simulink model "case6"  (R2024b)
settings: Solver=FixedStepAuto  StartTime=0  StopTime=1  FixedStep=1e-7  RelTol=1e-3
values from neighbouring files (symbols this model uses):
  SG_D_1_D = 0.01056    [IEEE9_case_parameters.m]    (also in case1_parameters.m; case2_parameters.m; case3_parameters.m; case4_parameters.m)
  SG_D_1_EnableSaturation = 0    [IEEE9_case_parameters.m]    (also in case1_parameters.m; case2_parameters.m; case3_parameters.m; case4_parameters.m)
  SG_D_1_f0 = 60    [IEEE9_case_parameters.m]    (also in case1_parameters.m; case2_parameters.m; case3_parameters.m; case4_parameters.m)
  SG_D_1_H = 7.5    [IEEE9_case_parameters.m]    (also in case1_parameters.m; case2_parameters.m; case3_parameters.m; case4_parameters.m)
  SG_D_1_K_A = 20    [IEEE9_case_parameters.m]    (also in case1_parameters.m; case2_parameters.m; case3_parameters.m; case4_parameters.m)
  SG_D_1_K_E = 1.000000e+1    (= 10)    [IEEE9_case_parameters.m]    (also in case1_parameters.m; case2_parameters.m; case3_parameters.m; case4_parameters.m)
  SG_D_1_K_F = 2.363    [IEEE9_case_parameters.m]    (also in case1_parameters.m; case2_parameters.m; case3_parameters.m; case4_parameters.m)
  SG_D_1_K_s = 0.5    [IEEE9_case_parameters.m]    (also in case1_parameters.m = 5; case2_parameters.m = 5; case3_parameters.m = 5; case4_parameters.m = 5)
  SG_D_1_R_a = 0.001088    [IEEE9_case_parameters.m]    (also in case1_parameters.m; case2_parameters.m; case3_parameters.m; case4_parameters.m)
  SG_D_1_S_A = 1    [IEEE9_case_parameters.m]    (also in case1_parameters.m; case2_parameters.m; case3_parameters.m; case4_parameters.m)
  SG_D_1_S_B = 0.103    [IEEE9_case_parameters.m]    (also in case1_parameters.m; case2_parameters.m; case3_parameters.m; case4_parameters.m)
  SG_D_1_S_N = 10.659857    [IEEE9_case_parameters.m]    (also in case1_parameters.m; case2_parameters.m; case3_parameters.m; case4_parameters.m)
  SG_D_1_SpeedPara = 200    [IEEE9_case_parameters.m]    (also in case1_parameters.m; case2_parameters.m; case3_parameters.m; case4_parameters.m)
  SG_D_1_T_0 = 0.720173    [IEEE9_case_parameters.m]    (also in case1_parameters.m = 0.755522; case2_parameters.m = 0.808931; case3_parameters.m = 0.869402; case4_parameters.m = 0.729316)
  SG_D_1_T_1 = 0.3    [IEEE9_case_parameters.m]    (also in case1_parameters.m; case2_parameters.m; case3_parameters.m; case4_parameters.m)
  SG_D_1_T_2 = 0.05    [IEEE9_case_parameters.m]    (also in case1_parameters.m; case2_parameters.m; case3_parameters.m; case4_parameters.m)
  SG_D_1_T_3 = 0.02    [IEEE9_case_parameters.m]    (also in case1_parameters.m; case2_parameters.m; case3_parameters.m; case4_parameters.m)
  SG_D_1_T_4 = 0.005    [IEEE9_case_parameters.m]    (also in case1_parameters.m; case2_parameters.m; case3_parameters.m; case4_parameters.m)
  SG_D_1_T_A = 0.02    [IEEE9_case_parameters.m]    (also in case1_parameters.m; case2_parameters.m; case3_parameters.m; case4_parameters.m)
  SG_D_1_T_dd = 8.000000e+0    (= 8)    [IEEE9_case_parameters.m]    (also in case1_parameters.m; case2_parameters.m; case3_parameters.m; case4_parameters.m)
  SG_D_1_T_ddd = 0.04    [IEEE9_case_parameters.m]    (also in case1_parameters.m; case2_parameters.m; case3_parameters.m; case4_parameters.m)
  SG_D_1_T_E = 0.314    [IEEE9_case_parameters.m]    (also in case1_parameters.m; case2_parameters.m; case3_parameters.m; case4_parameters.m)
  SG_D_1_T_F = 0.35    [IEEE9_case_parameters.m]    (also in case1_parameters.m; case2_parameters.m; case3_parameters.m; case4_parameters.m)
  SG_D_1_T_qd = 0.8    [IEEE9_case_parameters.m]    (also in case1_parameters.m; case2_parameters.m; case3_parameters.m; case4_parameters.m)
  SG_D_1_T_qdd = 0.02    [IEEE9_case_parameters.m]    (also in case1_parameters.m; case2_parameters.m; case3_parameters.m; case4_parameters.m)
  SG_D_1_T_speed = 0.1    [IEEE9_case_parameters.m]    (also in case1_parameters.m = 200; case2_parameters.m = 200; case3_parameters.m = 200; case4_parameters.m = 200)
  SG_D_1_T_w = 0.5    [IEEE9_case_parameters.m]    (also in case1_parameters.m; case2_parameters.m; case3_parameters.m; case4_parameters.m)
  SG_D_1_V_ref = 1.990276    [IEEE9_case_parameters.m]    (also in case1_parameters.m = 2.042296; case2_parameters.m = 2.051388; case3_parameters.m = 2.089584; case4_parameters.m = 2.01845)
  SG_D_1_w_ref = 376.991118    [IEEE9_case_parameters.m]    (also in case1_parameters.m; case2_parameters.m; case3_parameters.m; case4_parameters.m)
  SG_D_1_wb = 6.000000e+1    (= 60)    [IEEE9_case_parameters.m]    (also in case1_parameters.m; case2_parameters.m; case3_parameters.m; case4_parameters.m)
  SG_D_1_x_d = 1.9    [IEEE9_case_parameters.m]    (also in case1_parameters.m; case2_parameters.m; case3_parameters.m; case4_parameters.m)
  SG_D_1_x_dd = 0.302    [IEEE9_case_parameters.m]    (also in case1_parameters.m; case2_parameters.m; case3_parameters.m; case4_parameters.m)
  SG_D_1_x_ddd = 0.204    [IEEE9_case_parameters.m]    (also in case1_parameters.m; case2_parameters.m; case3_parameters.m; case4_parameters.m)
  SG_D_1_x_l = 0.05    [IEEE9_case_parameters.m]    (also in case1_parameters.m; case2_parameters.m; case3_parameters.m; case4_parameters.m)
  SG_D_1_x_q = 1.3    [IEEE9_case_parameters.m]    (also in case1_parameters.m; case2_parameters.m; case3_parameters.m; case4_parameters.m)
  SG_D_1_x_qd = 0.5    [IEEE9_case_parameters.m]    (also in case1_parameters.m; case2_parameters.m; case3_parameters.m; case4_parameters.m)
  SG_D_1_x_qdd = 0.3    [IEEE9_case_parameters.m]    (also in case1_parameters.m; case2_parameters.m; case3_parameters.m; case4_parameters.m)
  SG_D_2_D = 0.02    [IEEE9_case_parameters.m]    (also in case1_parameters.m; case2_parameters.m; case3_parameters.m; case4_parameters.m)
  SG_D_2_EnableSaturation = 0    [IEEE9_case_parameters.m]    (also in case1_parameters.m; case2_parameters.m; case3_parameters.m; case4_parameters.m)
  SG_D_2_f0 = 60    [IEEE9_case_parameters.m]    (also in case1_parameters.m; case2_parameters.m; case3_parameters.m; case4_parameters.m)
  SG_D_2_H = 8.000000e+0    (= 8)    [IEEE9_case_parameters.m]    (also in case1_parameters.m; case2_parameters.m; case3_parameters.m; case4_parameters.m)
  SG_D_2_K_A = 20    [IEEE9_case_parameters.m]    (also in case1_parameters.m; case2_parameters.m; case3_parameters.m; case4_parameters.m)
  SG_D_2_K_E = 1.000000e+1    (= 10)    [IEEE9_case_parameters.m]    (also in case1_parameters.m; case2_parameters.m; case3_parameters.m; case4_parameters.m)
  SG_D_2_K_F = 2.363    [IEEE9_case_parameters.m]    (also in case1_parameters.m; case2_parameters.m; case3_parameters.m; case4_parameters.m)
  SG_D_2_K_s = 0.5    [IEEE9_case_parameters.m]    (also in case1_parameters.m = 4; case2_parameters.m = 4; case3_parameters.m = 4; case4_parameters.m = 4)
  SG_D_2_R_a = 0.001088    [IEEE9_case_parameters.m]    (also in case1_parameters.m; case2_parameters.m; case3_parameters.m; case4_parameters.m)
  SG_D_2_S_A = 1    [IEEE9_case_parameters.m]    (also in case1_parameters.m; case2_parameters.m; case3_parameters.m; case4_parameters.m)
  SG_D_2_S_B = 0.103    [IEEE9_case_parameters.m]    (also in case1_parameters.m; case2_parameters.m; case3_parameters.m; case4_parameters.m)
  SG_D_2_S_N = 10.659857    [IEEE9_case_parameters.m]    (also in case1_parameters.m; case2_parameters.m; case3_parameters.m; case4_parameters.m)
  SG_D_2_SpeedPara = 200    [IEEE9_case_parameters.m]    (also in case1_parameters.m; case2_parameters.m; case3_parameters.m; case4_parameters.m)
  SG_D_2_T_0 = 1.632913    [IEEE9_case_parameters.m]    (also in case1_parameters.m = 1.632925; case2_parameters.m = 1.632915; case3_parameters.m = 1.632914; case4_parameters.m = 1.632927)
  SG_D_2_T_1 = 0.2    [IEEE9_case_parameters.m]    (also in case1_parameters.m; case2_parameters.m; case3_parameters.m; case4_parameters.m)
  SG_D_2_T_2 = 0.05    [IEEE9_case_parameters.m]    (also in case1_parameters.m; case2_parameters.m; case3_parameters.m; case4_parameters.m)
  SG_D_2_T_3 = 0.02    [IEEE9_case_parameters.m]    (also in case1_parameters.m; case2_parameters.m; case3_parameters.m; case4_parameters.m)
  SG_D_2_T_4 = 0.005    [IEEE9_case_parameters.m]    (also in case1_parameters.m; case2_parameters.m; case3_parameters.m; case4_parameters.m)
  SG_D_2_T_A = 0.02    [IEEE9_case_parameters.m]    (also in case1_parameters.m; case2_parameters.m; case3_parameters.m; case4_parameters.m)
  SG_D_2_T_dd = 7.9    [IEEE9_case_parameters.m]    (also in case1_parameters.m; case2_parameters.m; case3_parameters.m; case4_parameters.m)
  SG_D_2_T_ddd = 0.04    [IEEE9_case_parameters.m]    (also in case1_parameters.m; case2_parameters.m; case3_parameters.m; case4_parameters.m)
  SG_D_2_T_E = 0.314    [IEEE9_case_parameters.m]    (also in case1_parameters.m; case2_parameters.m; case3_parameters.m; case4_parameters.m)
  SG_D_2_T_F = 0.35    [IEEE9_case_parameters.m]    (also in case1_parameters.m; case2_parameters.m; case3_parameters.m; case4_parameters.m)
  SG_D_2_T_qd = 0.8    [IEEE9_case_parameters.m]    (also in case1_parameters.m; case2_parameters.m; case3_parameters.m; case4_parameters.m)
  SG_D_2_T_qdd = 0.015    [IEEE9_case_parameters.m]    (also in case1_parameters.m; case2_parameters.m; case3_parameters.m; case4_parameters.m)
  SG_D_2_T_speed = 0.1    [IEEE9_case_parameters.m]    (also in case1_parameters.m = 150; case2_parameters.m = 150; case3_parameters.m = 150; case4_parameters.m = 150)
  SG_D_2_T_w = 0.35    [IEEE9_case_parameters.m]    (also in case1_parameters.m; case2_parameters.m; case3_parameters.m; case4_parameters.m)
  SG_D_2_V_ref = 2.58547    [IEEE9_case_parameters.m]    (also in case1_parameters.m = 2.597896; case2_parameters.m = 2.587136; case3_parameters.m = 2.586042; case4_parameters.m = 2.599679)
  SG_D_2_w_ref = 376.991118    [IEEE9_case_parameters.m]    (also in case1_parameters.m; case2_parameters.m; case3_parameters.m; case4_parameters.m)
  SG_D_2_wb = 6.000000e+1    (= 60)    [IEEE9_case_parameters.m]    (also in case1_parameters.m; case2_parameters.m; case3_parameters.m; case4_parameters.m)
  SG_D_2_x_d = 1.8    [IEEE9_case_parameters.m]    (also in case1_parameters.m; case2_parameters.m; case3_parameters.m; case4_parameters.m)
  SG_D_2_x_dd = 0.302    [IEEE9_case_parameters.m]    (also in case1_parameters.m; case2_parameters.m; case3_parameters.m; case4_parameters.m)
  SG_D_2_x_ddd = 0.204    [IEEE9_case_parameters.m]    (also in case1_parameters.m; case2_parameters.m; case3_parameters.m; case4_parameters.m)
  SG_D_2_x_l = 0.05    [IEEE9_case_parameters.m]    (also in case1_parameters.m; case2_parameters.m; case3_parameters.m; case4_parameters.m)
  SG_D_2_x_q = 1.25    [IEEE9_case_parameters.m]    (also in case1_parameters.m; case2_parameters.m; case3_parameters.m; case4_parameters.m)
  SG_D_2_x_qd = 0.5    [IEEE9_case_parameters.m]    (also in case1_parameters.m; case2_parameters.m; case3_parameters.m; case4_parameters.m)
  SG_D_2_x_qdd = 0.3    [IEEE9_case_parameters.m]    (also in case1_parameters.m; case2_parameters.m; case3_parameters.m; case4_parameters.m)
  SG_D_3_D = 0.02    [IEEE9_case_parameters.m]    (also in case1_parameters.m; case2_parameters.m; case3_parameters.m; case4_parameters.m)
  SG_D_3_EnableSaturation = 0    [IEEE9_case_parameters.m]    (also in case1_parameters.m; case2_parameters.m; case3_parameters.m; case4_parameters.m)
  SG_D_3_f0 = 60    [IEEE9_case_parameters.m]    (also in case1_parameters.m; case2_parameters.m; case3_parameters.m; case4_parameters.m)
  SG_D_3_H = 7.7    [IEEE9_case_parameters.m]    (also in case1_parameters.m; case2_parameters.m; case3_parameters.m; case4_parameters.m)
  SG_D_3_K_A = 20    [IEEE9_case_parameters.m]    (also in case1_parameters.m; case2_parameters.m; case3_parameters.m; case4_parameters.m)
  SG_D_3_K_E = 1.000000e+1    (= 10)    [IEEE9_case_parameters.m]    (also in case1_parameters.m; case2_parameters.m; case3_parameters.m; case4_parameters.m)
  SG_D_3_K_F = 2.363    [IEEE9_case_parameters.m]    (also in case1_parameters.m; case2_parameters.m; case3_parameters.m; case4_parameters.m)
  SG_D_3_K_s = 0.2    [IEEE9_case_parameters.m]    (also in case1_parameters.m = 2; case2_parameters.m = 2; case3_parameters.m = 2; case4_parameters.m = 2)
  SG_D_3_R_a = 0.001088    [IEEE9_case_parameters.m]    (also in case1_parameters.m; case2_parameters.m; case3_parameters.m; case4_parameters.m)
  SG_D_3_S_A = 1    [IEEE9_case_parameters.m]    (also in case1_parameters.m; case2_parameters.m; case3_parameters.m; case4_parameters.m)
  SG_D_3_S_B = 0.103    [IEEE9_case_parameters.m]    (also in case1_parameters.m; case2_parameters.m; case3_parameters.m; case4_parameters.m)
  SG_D_3_S_N = 10.659857    [IEEE9_case_parameters.m]    (also in case1_parameters.m; case2_parameters.m; case3_parameters.m; case4_parameters.m)
  SG_D_3_SpeedPara = 200    [IEEE9_case_parameters.m]    (also in case1_parameters.m; case2_parameters.m; case3_parameters.m; case4_parameters.m)
  SG_D_3_T_0 = 0.850788    [IEEE9_case_parameters.m]    (also in case1_parameters.m = 0.850786; case2_parameters.m = 0.850787; case3_parameters.m; case4_parameters.m = 0.850786)
  SG_D_3_T_1 = 0.2    [IEEE9_case_parameters.m]    (also in case1_parameters.m; case2_parameters.m; case3_parameters.m; case4_parameters.m)
  SG_D_3_T_2 = 0.05    [IEEE9_case_parameters.m]    (also in case1_parameters.m; case2_parameters.m; case3_parameters.m; case4_parameters.m)
  SG_D_3_T_3 = 0.02    [IEEE9_case_parameters.m]    (also in case1_parameters.m; case2_parameters.m; case3_parameters.m; case4_parameters.m)
  SG_D_3_T_4 = 0.005    [IEEE9_case_parameters.m]    (also in case1_parameters.m; case2_parameters.m; case3_parameters.m; case4_parameters.m)
  SG_D_3_T_A = 0.02    [IEEE9_case_parameters.m]    (also in case1_parameters.m; case2_parameters.m; case3_parameters.m; case4_parameters.m)
  SG_D_3_T_dd = 8.1    [IEEE9_case_parameters.m]    (also in case1_parameters.m; case2_parameters.m; case3_parameters.m; case4_parameters.m)
  SG_D_3_T_ddd = 0.04    [IEEE9_case_parameters.m]    (also in case1_parameters.m; case2_parameters.m; case3_parameters.m; case4_parameters.m)
  SG_D_3_T_E = 0.314    [IEEE9_case_parameters.m]    (also in case1_parameters.m; case2_parameters.m; case3_parameters.m; case4_parameters.m)
  SG_D_3_T_F = 0.35    [IEEE9_case_parameters.m]    (also in case1_parameters.m; case2_parameters.m; case3_parameters.m; case4_parameters.m)
  SG_D_3_T_qd = 0.8    [IEEE9_case_parameters.m]    (also in case1_parameters.m; case2_parameters.m; case3_parameters.m; case4_parameters.m)
  SG_D_3_T_qdd = 0.015    [IEEE9_case_parameters.m]    (also in case1_parameters.m; case2_parameters.m; case3_parameters.m; case4_parameters.m)
  SG_D_3_T_speed = 0.1    [IEEE9_case_parameters.m]    (also in case1_parameters.m = 180; case2_parameters.m = 180; case3_parameters.m = 180; case4_parameters.m = 180)
  SG_D_3_T_w = 0.4    [IEEE9_case_parameters.m]    (also in case1_parameters.m; case2_parameters.m; case3_parameters.m; case4_parameters.m)
  SG_D_3_V_ref = 1.892727    [IEEE9_case_parameters.m]    (also in case1_parameters.m = 1.906439; case2_parameters.m = 1.895535; case3_parameters.m = 1.892105; case4_parameters.m = 1.906598)
  SG_D_3_w_ref = 376.991118    [IEEE9_case_parameters.m]    (also in case1_parameters.m; case2_parameters.m; case3_parameters.m; case4_parameters.m)
  SG_D_3_wb = 6.000000e+1    (= 60)    [IEEE9_case_parameters.m]    (also in case1_parameters.m; case2_parameters.m; case3_parameters.m; case4_parameters.m)
  SG_D_3_x_d = 1.85    [IEEE9_case_parameters.m]    (also in case1_parameters.m; case2_parameters.m; case3_parameters.m; case4_parameters.m)
  SG_D_3_x_dd = 0.302    [IEEE9_case_parameters.m]    (also in case1_parameters.m; case2_parameters.m; case3_parameters.m; case4_parameters.m)
  SG_D_3_x_ddd = 0.204    [IEEE9_case_parameters.m]    (also in case1_parameters.m; case2_parameters.m; case3_parameters.m; case4_parameters.m)
  SG_D_3_x_l = 0.05    [IEEE9_case_parameters.m]    (also in case1_parameters.m; case2_parameters.m; case3_parameters.m; case4_parameters.m)
  SG_D_3_x_q = 1.2    [IEEE9_case_parameters.m]    (also in case1_parameters.m; case2_parameters.m; case3_parameters.m; case4_parameters.m)
  SG_D_3_x_qd = 0.5    [IEEE9_case_parameters.m]    (also in case1_parameters.m; case2_parameters.m; case3_parameters.m; case4_parameters.m)
  SG_D_3_x_qdd = 0.3    [IEEE9_case_parameters.m]    (also in case1_parameters.m; case2_parameters.m; case3_parameters.m; case4_parameters.m)
(part 11 of 12)

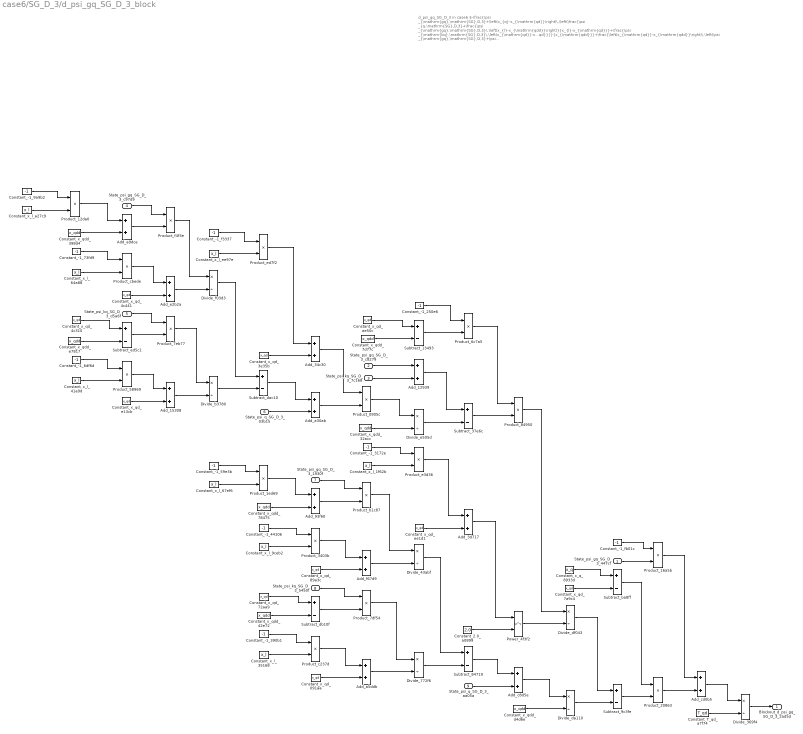
== system case6/SG_D_3/d_psi_gq_SG_D_3_block ==
  note: d_psi_gq_SG_D_3 in case6
      | $-\frac{\psi _{\mathrm{gq},\mathrm{SG},D,3}+\left(x_{q}-x_{\mathrm{qd}}\right)\,\left(\frac{\psi _{q,\mathrm{SG},D,3}+\frac{\psi _{\mathrm{gq},\mathrm{SG},D,3}\,\left(x_{l}-x_{\mathrm{qdd}}\right)}{x_{l}-x_{\mathrm{qd}}}+\frac{\psi _{\mathrm{kq},\mathrm{SG},D,3}\,\left(x_{\mathrm{qd}}-x_{\mathrm{qdd}}\right)}{x_{l}-x_{\mathrm{qd}}}}{x_{\mathrm{qdd}}}+\frac{\left(x_{\mathrm{qd}}-x_{\mathrm{qdd}}\right)\,\left(\psi _{\mathrm{gq},\mathrm{SG},D,3}+\psi _{\mathrm{kq},\mathrm{SG},D,3}+\frac{\left(x_{l}-x_{\mathrm{qd}}\right)\,\left(\psi _{q,\mathrm{SG},D,3}+\frac{\psi _{\mathrm{gq},\mathrm{SG},D,3}\,\left(x_{l}-x_{\mathrm{qdd}}\right)}{x_{l}-x_{\mathrm{qd}}}+\frac{\psi _{\mathrm{kq},\mathrm{SG},D,3}\,\left(x_{\mathrm{qd}}-x_{\mathrm{qdd}}\right)}{x_{l}-x_{\mathrm{qd}}}\right)}{x_{\mathrm{qdd}}}\right)}{{\left(x_{l}-x_{\mathrm{qd}}\right)}^2}\right)}{T_{\mathrm{qd}}}$
      | Automatically generated on 2025-10-31 19:19:17 .
  State_psi_gq_SG_D_3_447cf : Inport
  State_psi_gq_SG_D_3_c8279 : Inport  Port=2
  State_psi_kq_SG_D_3_7c168 : Inport  Port=3
  State_psi_gq_SG_D_3_c97d9 : Inport  Port=4
  State_psi_kq_SG_D_3_d5a6f : Inport  Port=5
  State_psi_q_SG_D_3_03b15 : Inport  Port=6
  State_psi_gq_SG_D_3_1930f : Inport  Port=7
  State_psi_kq_SG_D_3_5450f : Inport  Port=8
  State_psi_q_SG_D_3_aa05a : Inport  Port=9
  Add_12939 : Sum
  Add_15308 : Sum
  Add_34c30 : Sum
  Add_3d717 : Sum
  Add_93f60 : Sum
  Add_a30ab : Sum
  Add_a5ddb : Sum
  Add_a9dce : Sum
  Add_c8d5e : Sum
  Add_cd0b5 : Sum
  Add_e2b2a : Sum
  Add_f67d9 : Sum
  Constant_-1_250e6 : Constant  Value=-1
  Constant_-1_3172e : Constant  Value=-1
  Constant_-1_390b1 : Constant  Value=-1
  Constant_-1_44106 : Constant  Value=-1
  Constant_-1_59e3b : Constant  Value=-1
  Constant_-1_6df6d : Constant  Value=-1
  Constant_-1_73fd9 : Constant  Value=-1
  Constant_-1_9a9b2 : Constant  Value=-1
  Constant_-1_f3337 : Constant  Value=-1
  Constant_-1_fb01c : Constant  Value=-1
  Constant_2.0_a0899 : Constant  Value=2.0
  Constant_T_qd_a7f74 : Constant  Value=T_qd
  Constant_x_l_1f62b : Constant  Value=x_l
  Constant_x_l_35168 : Constant  Value=x_l
  Constant_x_l_41a9d : Constant  Value=x_l
  Constant_x_l_64a88 : Constant  Value=x_l
  Constant_x_l_67ef6 : Constant  Value=x_l
  Constant_x_l_9ceb2 : Constant  Value=x_l
  Constant_x_l_a27c9 : Constant  Value=x_l
  Constant_x_l_ee97e : Constant  Value=x_l
  Constant_x_q_8933d : Constant  Value=x_q
  Constant_x_qd_091aa : Constant  Value=x_qd
  Constant_x_qd_3e35b : Constant  Value=x_qd
  Constant_x_qd_4c310 : Constant  Value=x_qd
  Constant_x_qd_4c441 : Constant  Value=x_qd
  Constant_x_qd_72aa9 : Constant  Value=x_qd
  Constant_x_qd_7a9c4 : Constant  Value=x_qd
  Constant_x_qd_89a3c : Constant  Value=x_qd
  Constant_x_qd_ae50c : Constant  Value=x_qd
  Constant_x_qd_e13cb : Constant  Value=x_qd
  Constant_x_qd_ee1d1 : Constant  Value=x_qd
  Constant_x_qdd_32acc : Constant  Value=x_qdd
  Constant_x_qdd_398d4 : Constant  Value=x_qdd
  Constant_x_qdd_42e72 : Constant  Value=x_qdd
  Constant_x_qdd_78475 : Constant  Value=x_qdd
  Constant_x_qdd_7d77c : Constant  Value=x_qdd
  Constant_x_qdd_d4d6e : Constant  Value=x_qdd
  Constant_x_qdd_e7817 : Constant  Value=x_qdd
  Divide_369f4 : Product  Inputs=*/
  Divide_43abf : Product  Inputs=*/
  Divide_772f6 : Product  Inputs=*/
  Divide_b3780 : Product  Inputs=*/
  Divide_da110 : Product  Inputs=*/
  Divide_df043 : Product  Inputs=*/
  Divide_e505d : Product  Inputs=*/
  Divide_f03d3 : Product  Inputs=*/
  Power_4f3f2 : Math  Operator=pow
  Product_0905c : Product
  Product_12da0 : Product
  Product_16a5b : Product
  Product_1ed69 : Product
  Product_20863 : Product
  Product_3403b : Product
  Product_58969 : Product
  Product_6c7a5 : Product
  Product_7df54 : Product
  Product_7eb77 : Product
  Product_84950 : Product
  Product_b1c87 : Product
  Product_c237d : Product
  Product_cbede : Product
  Product_e3d36 : Product
  Product_ed7f2 : Product
  Product_f4f3e : Product
  Subtract_13493 : Sum  Inputs=+-
  Subtract_37e6c : Sum  Inputs=+-
  Subtract_84719 : Sum  Inputs=+-
  Subtract_9c3fe : Sum  Inputs=+-
  Subtract_ba8ff : Sum  Inputs=+-
  Subtract_dac10 : Sum  Inputs=+-
  Subtract_db10f : Sum  Inputs=+-
  Subtract_ed5c1 : Sum  Inputs=+-
  Blockout_d_psi_gq_SG_D_3_2ad5d : Outport
  wires:
  Constant_x_l_1f62b/1 -> Product_e3d36/2
  Constant_x_qd_4c310/1 -> Subtract_ed5c1/1
  Add_34c30/1 -> Product_0905c/1
  Constant_-1_9a9b2/1 -> Product_12da0/1
  Add_a9dce/1 -> Product_f4f3e/2
  Constant_x_qdd_e7817/1 -> Subtract_ed5c1/2
  Constant_x_qd_3e35b/1 -> Add_34c30/2
  Constant_x_l_a27c9/1 -> Product_12da0/2
  Constant_x_l_64a88/1 -> Product_cbede/2
  Add_a5ddb/1 -> Divide_772f6/2
  State_psi_kq_SG_D_3_7c168/1 -> Add_12939/2
  Constant_x_qdd_398d4/1 -> Add_a9dce/2
  Product_12da0/1 -> Add_a9dce/1
  Constant_x_qd_091aa/1 -> Add_a5ddb/2
  Product_6c7a5/1 -> Product_84950/1
  Constant_-1_59e3b/1 -> Product_1ed69/1
  Constant_-1_73fd9/1 -> Product_cbede/1
  Constant_-1_6df6d/1 -> Product_58969/1
  Constant_x_l_41a9d/1 -> Product_58969/2
  Constant_-1_250e6/1 -> Product_6c7a5/1
  Constant_-1_fb01c/1 -> Product_16a5b/1
  State_psi_gq_SG_D_3_c97d9/1 -> Product_f4f3e/1
  Product_1ed69/1 -> Add_93f60/1
  Product_cbede/1 -> Add_e2b2a/1
  Product_c237d/1 -> Add_a5ddb/1
  Constant_x_qd_4c441/1 -> Add_e2b2a/2
  Constant_-1_44106/1 -> Product_3403b/1
  State_psi_kq_SG_D_3_d5a6f/1 -> Product_7eb77/1
  Subtract_ed5c1/1 -> Product_7eb77/2
  Product_58969/1 -> Add_15308/1
  Add_93f60/1 -> Product_b1c87/2
  Add_e2b2a/1 -> Divide_f03d3/2
  Constant_x_qd_e13cb/1 -> Add_15308/2
  Product_f4f3e/1 -> Divide_f03d3/1
  Constant_T_qd_a7f74/1 -> Divide_369f4/2
  Product_3403b/1 -> Add_f67d9/1
  Product_7eb77/1 -> Divide_b3780/1
  Product_7df54/1 -> Divide_772f6/1
  Add_15308/1 -> Divide_b3780/2
  Constant_-1_f3337/1 -> Product_ed7f2/1
  Constant_x_qdd_32acc/1 -> Divide_e505d/2
  Constant_x_l_ee97e/1 -> Product_ed7f2/2
  Divide_f03d3/1 -> Subtract_dac10/1
  Constant_x_qd_7a9c4/1 -> Subtract_ba8ff/2
  Add_f67d9/1 -> Divide_43abf/2
  Divide_b3780/1 -> Subtract_dac10/2
  Constant_x_l_67ef6/1 -> Product_1ed69/2
  Product_ed7f2/1 -> Add_34c30/1
  Constant_-1_3172e/1 -> Product_e3d36/1
  Constant_x_l_9ceb2/1 -> Product_3403b/2
  Subtract_dac10/1 -> Add_a30ab/1
  State_psi_q_SG_D_3_03b15/1 -> Add_a30ab/2
  Constant_-1_390b1/1 -> Product_c237d/1
  Constant_x_qdd_78475/1 -> Add_93f60/2
  Constant_x_qd_72aa9/1 -> Subtract_db10f/1
  Constant_x_qdd_42e72/1 -> Subtract_db10f/2
  Constant_x_l_35168/1 -> Product_c237d/2
  Add_a30ab/1 -> Product_0905c/2
  Constant_x_qdd_7d77c/1 -> Subtract_13493/2
  State_psi_gq_SG_D_3_1930f/1 -> Product_b1c87/1
  Constant_x_qd_89a3c/1 -> Add_f67d9/2
  Divide_df043/1 -> Subtract_9c3fe/1
  State_psi_kq_SG_D_3_5450f/1 -> Product_7df54/1
  Subtract_db10f/1 -> Product_7df54/2
  Constant_x_qd_ae50c/1 -> Subtract_13493/1
  State_psi_gq_SG_D_3_c8279/1 -> Add_12939/1
  Product_0905c/1 -> Divide_e505d/1
  Product_b1c87/1 -> Divide_43abf/1
  Subtract_13493/1 -> Product_6c7a5/2
  Add_12939/1 -> Subtract_37e6c/1
  Divide_e505d/1 -> Subtract_37e6c/2
  Product_e3d36/1 -> Add_3d717/1
  Constant_x_qd_ee1d1/1 -> Add_3d717/2
  Divide_43abf/1 -> Subtract_84719/1
  Divide_772f6/1 -> Subtract_84719/2
  Subtract_37e6c/1 -> Product_84950/2
  Add_3d717/1 -> Power_4f3f2/1
  Constant_2.0_a0899/1 -> Power_4f3f2/2
  Subtract_84719/1 -> Add_c8d5e/1
  State_psi_q_SG_D_3_aa05a/1 -> Add_c8d5e/2
  Product_84950/1 -> Divide_df043/1
  Power_4f3f2/1 -> Divide_df043/2
  Add_c8d5e/1 -> Divide_da110/1
  Constant_x_qdd_d4d6e/1 -> Divide_da110/2
  Constant_x_q_8933d/1 -> Subtract_ba8ff/1
  Divide_da110/1 -> Subtract_9c3fe/2
  State_psi_gq_SG_D_3_447cf/1 -> Product_16a5b/2
  Subtract_ba8ff/1 -> Product_20863/1
  Subtract_9c3fe/1 -> Product_20863/2
  Product_16a5b/1 -> Add_cd0b5/1
  Product_20863/1 -> Add_cd0b5/2
  Add_cd0b5/1 -> Divide_369f4/1
  Divide_369f4/1 -> Blockout_d_psi_gq_SG_D_3_2ad5d/1

== system case6/SG_D_3/d_psi_kq_SG_D_3_block ==
  note: d_psi_kq_SG_D_3 in case6
      | $-\frac{\psi _{\mathrm{gq},\mathrm{SG},D,3}+\psi _{\mathrm{kq},\mathrm{SG},D,3}+\frac{\left(x_{l}-x_{\mathrm{qd}}\right)\,\left(\psi _{q,\mathrm{SG},D,3}+\frac{\psi _{\mathrm{gq},\mathrm{SG},D,3}\,\left(x_{l}-x_{\mathrm{qdd}}\right)}{x_{l}-x_{\mathrm{qd}}}+\frac{\psi _{\mathrm{kq},\mathrm{SG},D,3}\,\left(x_{\mathrm{qd}}-x_{\mathrm{qdd}}\right)}{x_{l}-x_{\mathrm{qd}}}\right)}{x_{\mathrm{qdd}}}}{T_{\mathrm{qdd}}}$
      | Automatically generated on 2025-10-31 19:19:21 .
  State_psi_gq_SG_D_3_3c968 : Inport
  State_psi_kq_SG_D_3_3550c : Inport  Port=2
  State_psi_gq_SG_D_3_f59cb : Inport  Port=3
  State_psi_kq_SG_D_3_48ef7 : Inport  Port=4
  State_psi_q_SG_D_3_2ea7c : Inport  Port=5
  Add_13628 : Sum
  Add_20637 : Sum
  Add_9f267 : Sum
  Add_a93cc : Sum
  Add_beb3e : Sum
  Add_d8732 : Sum
  Constant_-1_156e6 : Constant  Value=-1
  Constant_-1_5e9c5 : Constant  Value=-1
  Constant_-1_91f7a : Constant  Value=-1
  Constant_-1_da3ff : Constant  Value=-1
  Constant_-1_f171e : Constant  Value=-1
  Constant_T_qdd_c61c0 : Constant  Value=T_qdd
  Constant_x_l_1047d : Constant  Value=x_l
  Constant_x_l_3ae0a : Constant  Value=x_l
  Constant_x_l_9f8e8 : Constant  Value=x_l
  Constant_x_l_b4688 : Constant  Value=x_l
  Constant_x_qd_0905a : Constant  Value=x_qd
  Constant_x_qd_132c0 : Constant  Value=x_qd
  Constant_x_qd_4efa9 : Constant  Value=x_qd
  Constant_x_qd_d7acd : Constant  Value=x_qd
  Constant_x_qdd_76578 : Constant  Value=x_qdd
  Constant_x_qdd_b57e8 : Constant  Value=x_qdd
  Constant_x_qdd_babf2 : Constant  Value=x_qdd
  Divide_10821 : Product  Inputs=*/
  Divide_59c15 : Product  Inputs=*/
  Divide_b33fe : Product  Inputs=*/
  Divide_e3776 : Product  Inputs=*/
  Product_13363 : Product
  Product_4261e : Product
  Product_59fdc : Product
  Product_92618 : Product
  Product_b511d : Product
  Product_e2e02 : Product
  Product_e47ab : Product
  Product_faf11 : Product
  Subtract_0efec : Sum  Inputs=+-
  Subtract_c2b4a : Sum  Inputs=+-
  Subtract_f68ea : Sum  Inputs=+-
  Blockout_d_psi_kq_SG_D_3_6fe0f : Outport
  wires:
  State_psi_q_SG_D_3_2ea7c/1 -> Add_13628/2
  Constant_-1_5e9c5/1 -> Product_b511d/1
  Constant_-1_156e6/1 -> Product_4261e/1
  Constant_-1_f171e/1 -> Product_13363/1
  Constant_x_l_1047d/1 -> Product_b511d/2
  Constant_x_qdd_babf2/1 -> Add_a93cc/2
  Product_e2e02/1 -> Add_20637/1
  Constant_x_l_3ae0a/1 -> Product_4261e/2
  Constant_x_qd_0905a/1 -> Subtract_c2b4a/1
  Product_4261e/1 -> Add_a93cc/1
  Constant_x_l_9f8e8/1 -> Product_92618/2
  Constant_x_qdd_76578/1 -> Subtract_c2b4a/2
  Constant_-1_da3ff/1 -> Product_e2e02/1
  Constant_x_l_b4688/1 -> Product_e2e02/2
  State_psi_gq_SG_D_3_f59cb/1 -> Product_faf11/1
  Add_a93cc/1 -> Product_faf11/2
  Add_13628/1 -> Product_59fdc/2
  Product_b511d/1 -> Add_d8732/1
  Constant_x_qd_132c0/1 -> Add_d8732/2
  State_psi_kq_SG_D_3_48ef7/1 -> Product_e47ab/1
  Subtract_c2b4a/1 -> Product_e47ab/2
  Add_d8732/1 -> Divide_b33fe/2
  Constant_x_qd_d7acd/1 -> Add_20637/2
  Product_faf11/1 -> Divide_b33fe/1
  Product_e47ab/1 -> Divide_10821/1
  Add_20637/1 -> Divide_10821/2
  Constant_-1_91f7a/1 -> Product_92618/1
  Divide_b33fe/1 -> Subtract_0efec/1
  Add_9f267/1 -> Divide_e3776/1
  Divide_10821/1 -> Subtract_0efec/2
  Divide_e3776/1 -> Blockout_d_psi_kq_SG_D_3_6fe0f/1
  Product_92618/1 -> Add_beb3e/1
  Constant_x_qd_4efa9/1 -> Add_beb3e/2
  Subtract_0efec/1 -> Add_13628/1
  State_psi_gq_SG_D_3_3c968/1 -> Product_13363/2
  Add_beb3e/1 -> Product_59fdc/1
  Constant_T_qdd_c61c0/1 -> Divide_e3776/2
  Product_13363/1 -> Subtract_f68ea/1
  State_psi_kq_SG_D_3_3550c/1 -> Subtract_f68ea/2
  Product_59fdc/1 -> Divide_59c15/1
  Constant_x_qdd_b57e8/1 -> Divide_59c15/2
  Subtract_f68ea/1 -> Add_9f267/1
  Divide_59c15/1 -> Add_9f267/2

== system case6/SG_D_3/d_psi_q_SG_D_3_block ==
  note: d_psi_q_SG_D_3 in case6
      | $2\,\pi \,f_{0}\,\left(v_{d,\mathrm{SG},D,3}\,\cos\left(\theta _{\mathrm{SG},D,3}\right)+v_{q,\mathrm{SG},D,3}\,\sin\left(\theta _{\mathrm{SG},D,3}\right)-\frac{R_{a}\,\left(\psi _{q,\mathrm{SG},D,3}+\frac{\psi _{\mathrm{gq},\mathrm{SG},D,3}\,\left(x_{l}-x_{\mathrm{qdd}}\right)}{x_{l}-x_{\mathrm{qd}}}+\frac{\psi _{\mathrm{kq},\mathrm{SG},D,3}\,\left(x_{\mathrm{qd}}-x_{\mathrm{qdd}}\right)}{x_{l}-x_{\mathrm{qd}}}\right)}{x_{\mathrm{qdd}}}-\frac{\psi _{d,\mathrm{SG},D,3}\,w_{\mathrm{SG},D,3}}{2\,f_{0}\,\pi }\right)$
      | Automatically generated on 2025-10-31 19:18:59 .
  State_psi_gq_SG_D_3_44472 : Inport
  State_psi_kq_SG_D_3_a31f2 : Inport  Port=2
  State_psi_q_SG_D_3_3f014 : Inport  Port=3
  Input_v_d_SG_D_3_e9461 : Inport  Port=4
  State_theta_SG_D_3_3efc2 : Inport  Port=5
  Input_v_q_SG_D_3_d5a90 : Inport  Port=6
  State_theta_SG_D_3_e3679 : Inport  Port=7
  State_psi_d_SG_D_3_960b3 : Inport  Port=8
  State_w_SG_D_3_8c018 : Inport  Port=9
  Add_02d73 : Sum
  Add_3103c : Sum
  Add_8a7a6 : Sum
  Add_b9382 : Sum
  Add_c36db : Sum
  Constant_-1_739e7 : Constant  Value=-1
  Constant_-1_b34a5 : Constant  Value=-1
  Constant_-1_e5c6c : Constant  Value=-1
  Constant_-2.0_83048 : Constant  Value=-2.0
  Constant_2.0_3fe72 : Constant  Value=2.0
  Constant_R_a_d1c7d : Constant  Value=R_a
  Constant_f0_02d55 : Constant  Value=f0
  Constant_f0_054a1 : Constant  Value=f0
  Constant_pi_7d6a3 : Constant  Value=pi
  Constant_pi_ed56b : Constant  Value=pi
  Constant_x_l_15983 : Constant  Value=x_l
  Constant_x_l_3eb4b : Constant  Value=x_l
  Constant_x_l_daef7 : Constant  Value=x_l
  Constant_x_qd_65832 : Constant  Value=x_qd
  Constant_x_qd_7332c : Constant  Value=x_qd
  Constant_x_qd_b3384 : Constant  Value=x_qd
  Constant_x_qdd_1628b : Constant  Value=x_qdd
  Constant_x_qdd_341ac : Constant  Value=x_qdd
  Constant_x_qdd_f3557 : Constant  Value=x_qdd
  Divide_1b0b8 : Product  Inputs=*/
  Divide_28c9d : Product  Inputs=*/
  Divide_39289 : Product  Inputs=*/
  Divide_aa057 : Product  Inputs=*/
  MathFunc_cos_f9ceb : Trigonometry  Operator=cos
  MathFunc_sin_8cffe : Trigonometry
  Product_262db : Product
  Product_4ef78 : Product
  Product_5c219 : Product
  Product_6bef6 : Product
  Product_76210 : Product
  Product_82413 : Product
  Product_c6627 : Product
  Product_cbe64 : Product
  Product_cd56f : Product
  Product_d3a60 : Product
  Product_d4924 : Product
  Product_d9336 : Product
  Product_f5a51 : Product
  Product_fddf4 : Product
  Subtract_1f664 : Sum  Inputs=+-
  Subtract_2575a : Sum  Inputs=+-
  Subtract_55639 : Sum  Inputs=+-
  Subtract_e78ca : Sum  Inputs=+-
  Blockout_d_psi_q_SG_D_3_c3e35 : Outport
  wires:
  Constant_x_qd_7332c/1 -> Subtract_e78ca/1
  Constant_pi_7d6a3/1 -> Product_4ef78/2
  Product_76210/1 -> Divide_1b0b8/1
  Constant_x_l_15983/1 -> Product_6bef6/2
  Constant_f0_02d55/1 -> Product_d9336/2
  State_w_SG_D_3_8c018/1 -> Product_cbe64/2
  Constant_-1_b34a5/1 -> Product_82413/1
  Constant_x_qdd_1628b/1 -> Add_c36db/2
  Input_v_d_SG_D_3_e9461/1 -> Product_5c219/1
  Constant_x_qdd_f3557/1 -> Subtract_e78ca/2
  Constant_x_l_3eb4b/1 -> Product_82413/2
  Divide_39289/1 -> Add_02d73/2
  Product_82413/1 -> Add_c36db/1
  Constant_2.0_3fe72/1 -> Product_4ef78/1
  Add_b9382/1 -> Product_76210/2
  Constant_-1_739e7/1 -> Product_6bef6/1
  Constant_x_qd_b3384/1 -> Add_8a7a6/2
  Constant_-1_e5c6c/1 -> Product_f5a51/1
  Subtract_55639/1 -> Subtract_2575a/1
  Constant_x_l_daef7/1 -> Product_f5a51/2
  Subtract_2575a/1 -> Add_02d73/1
  Constant_f0_054a1/1 -> Product_cd56f/2
  State_theta_SG_D_3_e3679/1 -> MathFunc_sin_8cffe/1
  Constant_x_qd_65832/1 -> Add_3103c/2
  State_psi_gq_SG_D_3_44472/1 -> Product_fddf4/1
  Add_c36db/1 -> Product_fddf4/2
  Product_4ef78/1 -> Product_cd56f/1
  Product_6bef6/1 -> Add_3103c/1
  State_psi_kq_SG_D_3_a31f2/1 -> Product_d4924/1
  Subtract_e78ca/1 -> Product_d4924/2
  Product_f5a51/1 -> Add_8a7a6/1
  MathFunc_sin_8cffe/1 -> Product_d3a60/2
  Product_fddf4/1 -> Divide_28c9d/1
  Product_cd56f/1 -> Divide_39289/2
  Add_3103c/1 -> Divide_28c9d/2
  Product_d4924/1 -> Divide_aa057/1
  Add_8a7a6/1 -> Divide_aa057/2
  Input_v_q_SG_D_3_d5a90/1 -> Product_d3a60/1
  Divide_28c9d/1 -> Subtract_1f664/1
  Subtract_1f664/1 -> Add_b9382/1
  Divide_aa057/1 -> Subtract_1f664/2
  Divide_1b0b8/1 -> Subtract_55639/1
  State_psi_q_SG_D_3_3f014/1 -> Add_b9382/2
  Product_d3a60/1 -> Subtract_2575a/2
  Constant_R_a_d1c7d/1 -> Product_76210/1
  State_theta_SG_D_3_3efc2/1 -> MathFunc_cos_f9ceb/1
  Constant_x_qdd_341ac/1 -> Divide_1b0b8/2
  MathFunc_cos_f9ceb/1 -> Product_5c219/2
  Constant_-2.0_83048/1 -> Product_c6627/1
  Product_5c219/1 -> Subtract_55639/2
  State_psi_d_SG_D_3_960b3/1 -> Product_cbe64/1
  Constant_pi_ed56b/1 -> Product_c6627/2
  Product_cbe64/1 -> Divide_39289/1
  Product_c6627/1 -> Product_d9336/1
  Product_d9336/1 -> Product_262db/1
  Add_02d73/1 -> Product_262db/2
  Product_262db/1 -> Blockout_d_psi_q_SG_D_3_c3e35/1

== system case6/SG_D_3/d_theta_SG_D_3_block ==
  note: d_theta_SG_D_3 in case6
      | $w_{\mathrm{SG},D,3}-2\,\pi \,f_{0}$
      | Automatically generated on 2025-10-31 19:19:30 .
  State_w_SG_D_3_8bed8 : Inport
  Add_22e45 : Sum
  Constant_-2.0_35397 : Constant  Value=-2.0
  Constant_f0_5caf3 : Constant  Value=f0
  Constant_pi_43b28 : Constant  Value=pi
  Product_6d06f : Product
  Product_9bda9 : Product
  Blockout_d_theta_SG_D_3_22a58 : Outport
  wires:
  Constant_-2.0_35397/1 -> Product_9bda9/1
  Constant_pi_43b28/1 -> Product_9bda9/2
  State_w_SG_D_3_8bed8/1 -> Add_22e45/2
  Product_9bda9/1 -> Product_6d06f/1
  Constant_f0_5caf3/1 -> Product_6d06f/2
  Product_6d06f/1 -> Add_22e45/1
  Add_22e45/1 -> Blockout_d_theta_SG_D_3_22a58/1

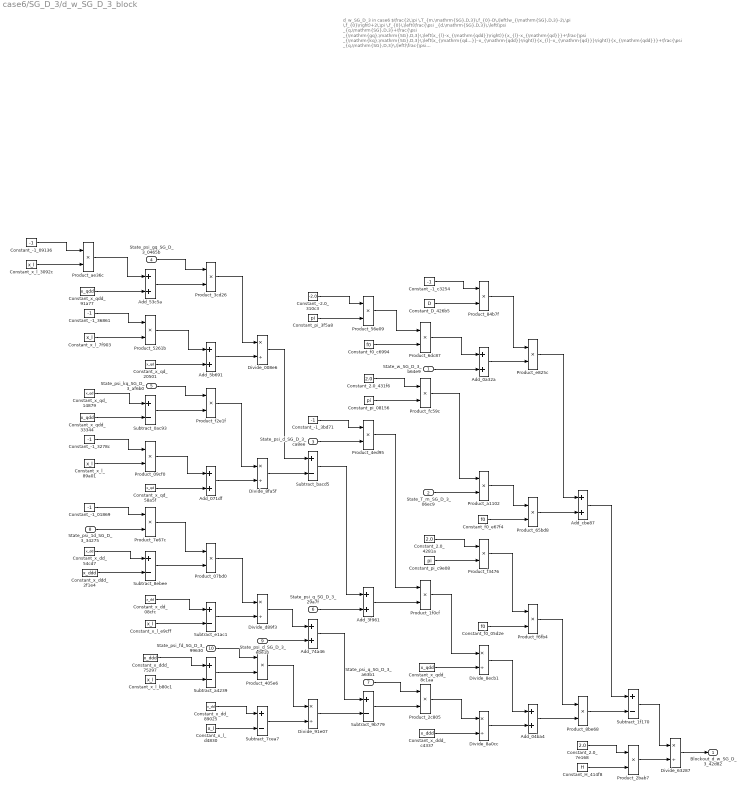
== system case6/SG_D_3/d_w_SG_D_3_block ==
  note: d_w_SG_D_3 in case6
      | $\frac{2\,\pi \,T_{m,\mathrm{SG},D,3}\,f_{0}-D\,\left(w_{\mathrm{SG},D,3}-2\,\pi \,f_{0}\right)+2\,\pi \,f_{0}\,\left(\frac{\psi _{d,\mathrm{SG},D,3}\,\left(\psi _{q,\mathrm{SG},D,3}+\frac{\psi _{\mathrm{gq},\mathrm{SG},D,3}\,\left(x_{l}-x_{\mathrm{qdd}}\right)}{x_{l}-x_{\mathrm{qd}}}+\frac{\psi _{\mathrm{kq},\mathrm{SG},D,3}\,\left(x_{\mathrm{qd}}-x_{\mathrm{qdd}}\right)}{x_{l}-x_{\mathrm{qd}}}\right)}{x_{\mathrm{qdd}}}+\frac{\psi _{q,\mathrm{SG},D,3}\,\left(\frac{\psi _{\mathrm{1d},\mathrm{SG},D,3}\,\left(x_{\mathrm{dd}}-x_{\mathrm{ddd}}\right)}{x_{\mathrm{dd}}-x_{l}}-\psi _{d,\mathrm{SG},D,3}+\frac{\psi _{\mathrm{fd},\mathrm{SG},D,3}\,\left(x_{\mathrm{ddd}}-x_{l}\right)}{x_{\mathrm{dd}}-x_{l}}\right)}{x_{\mathrm{ddd}}}\right)}{2\,H}$
      | Automatically generated on 2025-10-31 19:19:29 .
  State_w_SG_D_3_b64e9 : Inport
  State_T_m_SG_D_3_06ec9 : Inport  Port=2
  State_psi_d_SG_D_3_ca8ee : Inport  Port=3
  State_psi_gq_SG_D_3_0465b : Inport  Port=4
  State_psi_kq_SG_D_3_af6b0 : Inport  Port=5
  State_psi_q_SG_D_3_29a7f : Inport  Port=6
  State_psi_q_SG_D_3_a63b1 : Inport  Port=7
  State_psi_1d_SG_D_3_34275 : Inport  Port=8
  State_psi_d_SG_D_3_ebe1b : Inport  Port=9
  State_psi_fd_SG_D_3_99630 : Inport  Port=10
  Add_04ba4 : Sum
  Add_071df : Sum
  Add_0a32a : Sum
  Add_3f961 : Sum
  Add_53c5a : Sum
  Add_5b691 : Sum
  Add_74a46 : Sum
  Add_cbe87 : Sum
  Constant_-1_01869 : Constant  Value=-1
  Constant_-1_09136 : Constant  Value=-1
  Constant_-1_3278c : Constant  Value=-1
  Constant_-1_36861 : Constant  Value=-1
  Constant_-1_3bd71 : Constant  Value=-1
  Constant_-1_c3254 : Constant  Value=-1
  Constant_-2.0_310c3 : Constant  Value=-2.0
  Constant_2.0_4281a : Constant  Value=2.0
  Constant_2.0_431f6 : Constant  Value=2.0
  Constant_2.0_7e168 : Constant  Value=2.0
  Constant_D_426b5 : Constant  Value=D
  Constant_H_414f8 : Constant  Value=H
  Constant_f0_05d2e : Constant  Value=f0
  Constant_f0_c6994 : Constant  Value=f0
  Constant_f0_e67f4 : Constant  Value=f0
  Constant_pi_08156 : Constant  Value=pi
  Constant_pi_3f5a8 : Constant  Value=pi
  Constant_pi_c9e08 : Constant  Value=pi
  Constant_x_dd_08cfc : Constant  Value=x_dd
  Constant_x_dd_54cd7 : Constant  Value=x_dd
  Constant_x_dd_89025 : Constant  Value=x_dd
  Constant_x_ddd_2f1e4 : Constant  Value=x_ddd
  Constant_x_ddd_75297 : Constant  Value=x_ddd
  Constant_x_ddd_c4337 : Constant  Value=x_ddd
  Constant_x_l_3092c : Constant  Value=x_l
  Constant_x_l_7f903 : Constant  Value=x_l
  Constant_x_l_89a01 : Constant  Value=x_l
  Constant_x_l_b80c1 : Constant  Value=x_l
  Constant_x_l_d4830 : Constant  Value=x_l
  Constant_x_l_e9cff : Constant  Value=x_l
  Constant_x_qd_14879 : Constant  Value=x_qd
  Constant_x_qd_20501 : Constant  Value=x_qd
  Constant_x_qd_58a5f : Constant  Value=x_qd
  Constant_x_qdd_33344 : Constant  Value=x_qdd
  Constant_x_qdd_8c1aa : Constant  Value=x_qdd
  Constant_x_qdd_91a77 : Constant  Value=x_qdd
  Divide_008e6 : Product  Inputs=*/
  Divide_63287 : Product  Inputs=*/
  Divide_8a0cc : Product  Inputs=*/
  Divide_8ecb1 : Product  Inputs=*/
  Divide_8fa5f : Product  Inputs=*/
  Divide_91e07 : Product  Inputs=*/
  Divide_d89f3 : Product  Inputs=*/
  Product_07bd0 : Product
  Product_09cf0 : Product
  Product_1f0cf : Product
  Product_2bab7 : Product
  Product_2c805 : Product
  Product_3cd26 : Product
  Product_405e6 : Product
  Product_4ed95 : Product
  Product_5261b : Product
  Product_56e09 : Product
  Product_65bd8 : Product
  Product_6dc87 : Product
  Product_7e67c : Product
  Product_84b7f : Product
  Product_8be68 : Product
  Product_a1102 : Product
  Product_ae36c : Product
  Product_e825c : Product
  Product_f2e1f : Product
  Product_f3476 : Product
  Product_f6fb4 : Product
  Product_fc59c : Product
  Subtract_0ac93 : Sum  Inputs=+-
  Subtract_1f170 : Sum  Inputs=+-
  Subtract_7cea7 : Sum  Inputs=+-
  Subtract_8ebee : Sum  Inputs=+-
  Subtract_9b779 : Sum  Inputs=+-
  Subtract_a4239 : Sum  Inputs=+-
  Subtract_bacd5 : Sum  Inputs=+-
  Subtract_e1ac1 : Sum  Inputs=+-
  Blockout_d_w_SG_D_3_42d82 : Outport
  wires:
  Constant_x_qd_14879/1 -> Subtract_0ac93/1
  Subtract_8ebee/1 -> Product_07bd0/2
  Subtract_1f170/1 -> Divide_63287/1
  Constant_-1_09136/1 -> Product_ae36c/1
  Add_53c5a/1 -> Product_3cd26/2
  Constant_x_qdd_33344/1 -> Subtract_0ac93/2
  Subtract_a4239/1 -> Product_405e6/2
  Constant_x_l_3092c/1 -> Product_ae36c/2
  State_psi_d_SG_D_3_ebe1b/1 -> Add_74a46/2
  Add_5b691/1 -> Divide_008e6/2
  Constant_x_dd_08cfc/1 -> Subtract_e1ac1/1
  Constant_x_l_7f903/1 -> Product_5261b/2
  Constant_-1_c3254/1 -> Product_84b7f/1
  Divide_91e07/1 -> Subtract_9b779/2
  Constant_x_ddd_2f1e4/1 -> Subtract_8ebee/2
  Constant_x_qdd_91a77/1 -> Add_53c5a/2
  Constant_pi_08156/1 -> Product_fc59c/2
  Product_ae36c/1 -> Add_53c5a/1
  Constant_-2.0_310c3/1 -> Product_56e09/1
  Constant_-1_36861/1 -> Product_5261b/1
  Constant_2.0_4281a/1 -> Product_f3476/1
  Product_56e09/1 -> Product_6dc87/1
  Constant_-1_3278c/1 -> Product_09cf0/1
  Subtract_bacd5/1 -> Add_3f961/1
  Constant_x_l_89a01/1 -> Product_09cf0/2
  Constant_x_l_b80c1/1 -> Subtract_a4239/2
  Constant_-1_01869/1 -> Product_7e67c/1
  State_psi_1d_SG_D_3_34275/1 -> Product_7e67c/2
  Constant_x_dd_54cd7/1 -> Subtract_8ebee/1
  Product_7e67c/1 -> Product_07bd0/1
  State_psi_gq_SG_D_3_0465b/1 -> Product_3cd26/1
  Constant_x_qd_20501/1 -> Add_5b691/2
  Product_5261b/1 -> Add_5b691/1
  State_psi_kq_SG_D_3_af6b0/1 -> Product_f2e1f/1
  Subtract_0ac93/1 -> Product_f2e1f/2
  Product_f3476/1 -> Product_f6fb4/1
  Product_6dc87/1 -> Add_0a32a/1
  Product_09cf0/1 -> Add_071df/1
  State_psi_q_SG_D_3_a63b1/1 -> Product_2c805/1
  Constant_x_qd_58a5f/1 -> Add_071df/2
  Constant_x_l_e9cff/1 -> Subtract_e1ac1/2
  Constant_x_ddd_75297/1 -> Subtract_a4239/1
  Constant_x_l_d4830/1 -> Subtract_7cea7/2
  Product_3cd26/1 -> Divide_008e6/1
  Product_f2e1f/1 -> Divide_8fa5f/1
  Add_071df/1 -> Divide_8fa5f/2
  Product_07bd0/1 -> Divide_d89f3/1
  Subtract_e1ac1/1 -> Divide_d89f3/2
  Constant_2.0_431f6/1 -> Product_fc59c/1
  State_psi_fd_SG_D_3_99630/1 -> Product_405e6/1
  Constant_x_dd_89025/1 -> Subtract_7cea7/1
  Divide_008e6/1 -> Subtract_bacd5/1
  Product_405e6/1 -> Divide_91e07/1
  Divide_8fa5f/1 -> Subtract_bacd5/2
  Divide_d89f3/1 -> Add_74a46/1
  Product_8be68/1 -> Subtract_1f170/2
  Subtract_7cea7/1 -> Divide_91e07/2
  Constant_pi_3f5a8/1 -> Product_56e09/2
  Constant_pi_c9e08/1 -> Product_f3476/2
  Constant_-1_3bd71/1 -> Product_4ed95/1
  State_psi_d_SG_D_3_ca8ee/1 -> Product_4ed95/2
  State_psi_q_SG_D_3_29a7f/1 -> Add_3f961/2
  Add_74a46/1 -> Subtract_9b779/1
  Constant_f0_c6994/1 -> Product_6dc87/2
  Product_4ed95/1 -> Product_1f0cf/1
  Add_3f961/1 -> Product_1f0cf/2
  Subtract_9b779/1 -> Product_2c805/2
  Constant_D_426b5/1 -> Product_84b7f/2
  State_w_SG_D_3_b64e9/1 -> Add_0a32a/2
  Product_fc59c/1 -> Product_a1102/1
  State_T_m_SG_D_3_06ec9/1 -> Product_a1102/2
  Product_1f0cf/1 -> Divide_8ecb1/1
  Constant_x_qdd_8c1aa/1 -> Divide_8ecb1/2
  Product_2c805/1 -> Divide_8a0cc/1
  Constant_x_ddd_c4337/1 -> Divide_8a0cc/2
  Product_84b7f/1 -> Product_e825c/1
  Add_0a32a/1 -> Product_e825c/2
  Product_a1102/1 -> Product_65bd8/1
  Constant_f0_e67f4/1 -> Product_65bd8/2
  Constant_f0_05d2e/1 -> Product_f6fb4/2
  Divide_8ecb1/1 -> Add_04ba4/1
  Divide_8a0cc/1 -> Add_04ba4/2
  Product_e825c/1 -> Add_cbe87/1
  Product_65bd8/1 -> Add_cbe87/2
  Product_f6fb4/1 -> Product_8be68/1
  Add_04ba4/1 -> Product_8be68/2
  Add_cbe87/1 -> Subtract_1f170/1
  Constant_2.0_7e168/1 -> Product_2bab7/1
  Constant_H_414f8/1 -> Product_2bab7/2
  Product_2bab7/1 -> Divide_63287/2
  Divide_63287/1 -> Blockout_d_w_SG_D_3_42d82/1

== system case6/SG_D_3/i_d_SG_D_3_block ==
  note: i_d_SG_D_3 in case6
      | $\frac{\sin\left(\theta _{\mathrm{SG},D,3}\right)\,\left(\frac{\psi _{\mathrm{1d},\mathrm{SG},D,3}\,\left(x_{\mathrm{dd}}-x_{\mathrm{ddd}}\right)}{x_{\mathrm{dd}}-x_{l}}-\psi _{d,\mathrm{SG},D,3}+\frac{\psi _{\mathrm{fd},\mathrm{SG},D,3}\,\left(x_{\mathrm{ddd}}-x_{l}\right)}{x_{\mathrm{dd}}-x_{l}}\right)}{x_{\mathrm{ddd}}}-\frac{\cos\left(\theta _{\mathrm{SG},D,3}\right)\,\left(\psi _{q,\mathrm{SG},D,3}+\frac{\psi _{\mathrm{gq},\mathrm{SG},D,3}\,\left(x_{l}-x_{\mathrm{qdd}}\right)}{x_{l}-x_{\mathrm{qd}}}+\frac{\psi _{\mathrm{kq},\mathrm{SG},D,3}\,\left(x_{\mathrm{qd}}-x_{\mathrm{qdd}}\right)}{x_{l}-x_{\mathrm{qd}}}\right)}{x_{\mathrm{qdd}}}$
      | Automatically generated on 2025-10-31 19:19:57 .
  State_psi_gq_SG_D_3_f8709 : Inport
  State_psi_kq_SG_D_3_4574d : Inport  Port=2
  State_psi_q_SG_D_3_eb21b : Inport  Port=3
  State_theta_SG_D_3_5e6c6 : Inport  Port=4
  State_psi_1d_SG_D_3_699bf : Inport  Port=5
  State_psi_d_SG_D_3_b37a4 : Inport  Port=6
  State_psi_fd_SG_D_3_236ec : Inport  Port=7
  State_theta_SG_D_3_8c3e3 : Inport  Port=8
  Add_1a63d : Sum
  Add_213c4 : Sum
  Add_385ef : Sum
  Add_571fb : Sum
  Add_8c156 : Sum
  Constant_-1_0a65e : Constant  Value=-1
  Constant_-1_22060 : Constant  Value=-1
  Constant_-1_4bcb3 : Constant  Value=-1
  Constant_-1_6eafb : Constant  Value=-1
  Constant_-1_b62a3 : Constant  Value=-1
  Constant_x_dd_746eb : Constant  Value=x_dd
  Constant_x_dd_a5cee : Constant  Value=x_dd
  Constant_x_dd_da462 : Constant  Value=x_dd
  Constant_x_ddd_290b1 : Constant  Value=x_ddd
  Constant_x_ddd_8363c : Constant  Value=x_ddd
  Constant_x_ddd_cd99d : Constant  Value=x_ddd
  Constant_x_l_39b88 : Constant  Value=x_l
  Constant_x_l_4310e : Constant  Value=x_l
  Constant_x_l_4323d : Constant  Value=x_l
  Constant_x_l_80f2a : Constant  Value=x_l
  Constant_x_l_ac448 : Constant  Value=x_l
  Constant_x_l_b13a7 : Constant  Value=x_l
  Constant_x_qd_03e6e : Constant  Value=x_qd
  Constant_x_qd_075d2 : Constant  Value=x_qd
  Constant_x_qd_40460 : Constant  Value=x_qd
  Constant_x_qdd_0016f : Constant  Value=x_qdd
  Constant_x_qdd_3b7fb : Constant  Value=x_qdd
  Constant_x_qdd_5dd9c : Constant  Value=x_qdd
  Divide_6206e : Product  Inputs=*/
  Divide_940b9 : Product  Inputs=*/
  Divide_c3c5a : Product  Inputs=*/
  Divide_e0463 : Product  Inputs=*/
  Divide_f873b : Product  Inputs=*/
  Divide_ff13d : Product  Inputs=*/
  MathFunc_cos_6c771 : Trigonometry  Operator=cos
  MathFunc_sin_a2a3c : Trigonometry
  Product_159b1 : Product
  Product_1fca5 : Product
  Product_21e11 : Product
  Product_52a2b : Product
  Product_8341d : Product
  Product_88923 : Product
  Product_9cdb1 : Product
  Product_9e65c : Product
  Product_a310e : Product
  Product_e9213 : Product
  Product_fe4b6 : Product
  Subtract_201d8 : Sum  Inputs=+-
  Subtract_2311e : Sum  Inputs=+-
  Subtract_4043a : Sum  Inputs=+-
  Subtract_7e338 : Sum  Inputs=+-
  Subtract_97a47 : Sum  Inputs=+-
  Subtract_99040 : Sum  Inputs=+-
  Subtract_9e741 : Sum  Inputs=+-
  Subtract_af088 : Sum  Inputs=+-
  Blockout_i_d_SG_D_3_01a92 : Outport
  wires:
  Constant_x_qd_075d2/1 -> Subtract_97a47/1
  Subtract_2311e/1 -> Blockout_i_d_SG_D_3_01a92/1
  Constant_-1_b62a3/1 -> Product_88923/1
  Constant_x_l_4310e/1 -> Product_159b1/2
  Constant_x_qdd_5dd9c/1 -> Add_8c156/2
  Constant_x_qdd_0016f/1 -> Subtract_97a47/2
  Constant_x_l_b13a7/1 -> Product_88923/2
  Divide_e0463/1 -> Subtract_2311e/1
  Product_88923/1 -> Add_8c156/1
  Constant_x_ddd_cd99d/1 -> Subtract_201d8/2
  Constant_-1_6eafb/1 -> Product_159b1/1
  Constant_-1_0a65e/1 -> Product_52a2b/1
  Constant_x_l_ac448/1 -> Product_52a2b/2
  State_psi_1d_SG_D_3_699bf/1 -> Product_e9213/2
  State_psi_gq_SG_D_3_f8709/1 -> Product_9cdb1/1
  Product_e9213/1 -> Product_fe4b6/1
  Add_8c156/1 -> Product_9cdb1/2
  Product_159b1/1 -> Add_1a63d/1
  Constant_x_qd_03e6e/1 -> Add_1a63d/2
  State_psi_kq_SG_D_3_4574d/1 -> Product_1fca5/1
  Subtract_9e741/1 -> Divide_f873b/2
  Subtract_97a47/1 -> Product_1fca5/2
  Product_52a2b/1 -> Add_385ef/1
  Constant_x_ddd_290b1/1 -> Subtract_4043a/1
  Constant_x_qd_40460/1 -> Add_385ef/2
  Constant_-1_4bcb3/1 -> Product_e9213/1
  Constant_x_dd_746eb/1 -> Subtract_201d8/1
  Product_9cdb1/1 -> Divide_c3c5a/1
  Add_1a63d/1 -> Divide_c3c5a/2
  Product_1fca5/1 -> Divide_ff13d/1
  Add_385ef/1 -> Divide_ff13d/2
  Divide_f873b/1 -> Subtract_99040/2
  Subtract_201d8/1 -> Product_fe4b6/2
  State_theta_SG_D_3_5e6c6/1 -> MathFunc_cos_6c771/1
  Constant_x_dd_da462/1 -> Subtract_af088/1
  Product_9e65c/1 -> Product_a310e/1
  Constant_x_l_80f2a/1 -> Subtract_af088/2
  Add_213c4/1 -> Subtract_99040/1
  Constant_x_l_39b88/1 -> Subtract_4043a/2
  State_theta_SG_D_3_8c3e3/1 -> MathFunc_sin_a2a3c/1
  Divide_c3c5a/1 -> Subtract_7e338/1
  Add_571fb/1 -> Product_9e65c/2
  Divide_ff13d/1 -> Subtract_7e338/2
  Product_fe4b6/1 -> Divide_6206e/1
  Subtract_af088/1 -> Divide_6206e/2
  State_psi_fd_SG_D_3_236ec/1 -> Product_8341d/1
  Divide_940b9/1 -> Subtract_2311e/2
  Subtract_4043a/1 -> Product_8341d/2
  Constant_x_dd_a5cee/1 -> Subtract_9e741/1
  Subtract_7e338/1 -> Add_571fb/1
  Constant_x_l_4323d/1 -> Subtract_9e741/2
  Constant_-1_22060/1 -> Product_9e65c/1
  State_psi_q_SG_D_3_eb21b/1 -> Add_571fb/2
  Divide_6206e/1 -> Add_213c4/1
  State_psi_d_SG_D_3_b37a4/1 -> Add_213c4/2
  Product_8341d/1 -> Divide_f873b/1
  MathFunc_cos_6c771/1 -> Product_a310e/2
  MathFunc_sin_a2a3c/1 -> Product_21e11/2
  Subtract_99040/1 -> Product_21e11/1
  Product_a310e/1 -> Divide_e0463/1
  Constant_x_qdd_3b7fb/1 -> Divide_e0463/2
  Product_21e11/1 -> Divide_940b9/1
  Constant_x_ddd_8363c/1 -> Divide_940b9/2
